simulink model "trajectoryControlAnalysis"  (R2016b)
settings: Solver=VariableStepAuto  StartTime=0.0  StopTime=2  MaxStep=0.01  RelTol=1e-4  EnableMultiTasking=on
values from neighbouring files (symbols this model uses):
  La = 1    [analysis.m]    (also in main.m; purePursuitController.m = 0)
  v = 1    [analysis.m]    (also in main.m = U(1,inode))
undefined symbols (not defined in the file or in its folder): bic, g, gainK
settings Model: Creator=aniket  LastModifiedBy=aniket
settings DataIOCC: LimitDataPoints=on  SaveOutput=off  SaveTime=off
settings OptimizationCC: ExpressionDepthLimit=2147483647  LifeSpan=1
settings DebuggingCC: UnderspecifiedInitializationDetection=Classic  MergeDetectMultiDrivingBlocksExec=none  FcnCallInpInsideContextMsg=warning  AllowSymbolicDim=off  StateNameClashWarn=warning  SFUnexpectedBacktrackingDiag=warning  SFNoUnconditionalDefaultTransitionDiag=warning  SFExecutionAtInitializationDiag=none
settings GRTTargetCC: TargetLangStandard=C89/C90 (ANSI)  GeneratePreprocessorConditionals=Disable all  CombineOutputUpdateFcns=off  GRTInterface=on

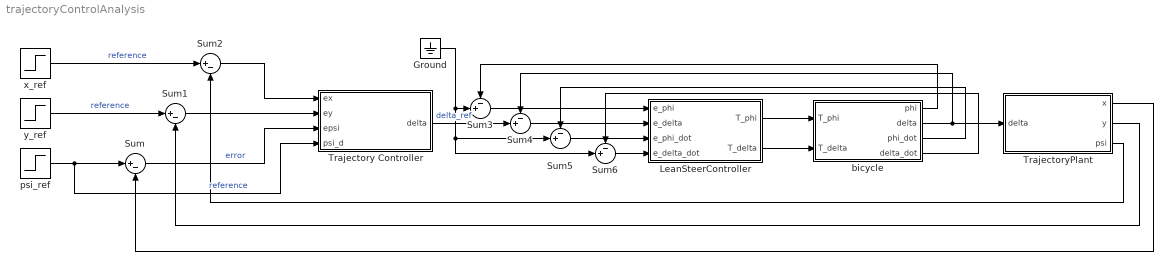
== system trajectoryControlAnalysis ==
  Ground : Ground
  LeanSteerController : Subsystem
  Sum : Sum  Inputs=|+-
  Sum1 : Sum  Inputs=|+-
  Sum2 : Sum  Inputs=|+-
  Sum{3..6} (4 alike) : Sum  Inputs=-+|
  Trajectory Controller : Subsystem
  TrajectoryPlant : Subsystem
  bicycle : Subsystem
  psi_ref : Step  SampleTime=0
  x_ref : Step  SampleTime=0
  y_ref : Step  SampleTime=0
  wires:
  psi_ref/1 -> Trajectory Controller/4(psi_d), Sum/1  "reference"
  TrajectoryPlant/1(x) -> Sum/2
  y_ref/1 -> Sum1/1  "reference"
  x_ref/1 -> Sum2/1  "reference"
  TrajectoryPlant/2(y) -> Sum1/2
  TrajectoryPlant/3(psi) -> Sum2/2
  Sum/1 -> Trajectory Controller/3(epsi)  "error"
  Sum1/1 -> Trajectory Controller/2(ey)
  Sum2/1 -> Trajectory Controller/1(ex)
  LeanSteerController/1(T_phi) -> bicycle/1(T_phi)
  LeanSteerController/2(T_delta) -> bicycle/2(T_delta)
  Sum3/1 -> LeanSteerController/1(e_phi)
  Sum4/1 -> LeanSteerController/2(e_delta)
  Sum5/1 -> LeanSteerController/3(e_phi_dot)
  Sum6/1 -> LeanSteerController/4(e_delta_dot)
  bicycle/1(phi) -> Sum3/1
  bicycle/2(delta) -> TrajectoryPlant/1(delta), Sum4/1
  bicycle/3(phi_dot) -> Sum5/1
  bicycle/4(delta_dot) -> Sum6/1
  Trajectory Controller/1(delta) -> Sum4/2  "delta_ref"
  Ground/1 -> Sum6/2, Sum5/2, Sum3/2

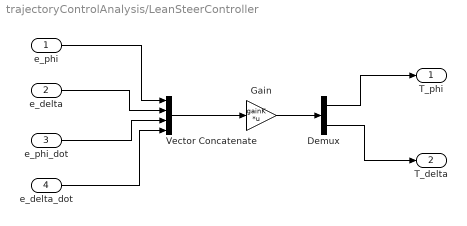
== system trajectoryControlAnalysis/LeanSteerController ==
  e_phi : Inport
  e_delta : Inport  Port=2
  e_phi_dot : Inport  Port=3
  e_delta_dot : Inport  Port=4
  Demux : Demux  Outputs=2
  Gain : Gain  Gain=gainK  Multiplication=Matrix(K*u) (u vector)
  Vector Concatenate : Concatenate  NumInputs=4
  T_phi : Outport
  T_delta : Outport  Port=2
  wires:
  Gain/1 -> Demux/1
  e_phi/1 -> Vector Concatenate/1
  e_delta/1 -> Vector Concatenate/2
  e_phi_dot/1 -> Vector Concatenate/3
  e_delta_dot/1 -> Vector Concatenate/4
  Vector Concatenate/1 -> Gain/1
  Demux/2 -> T_delta/1
  Demux/1 -> T_phi/1

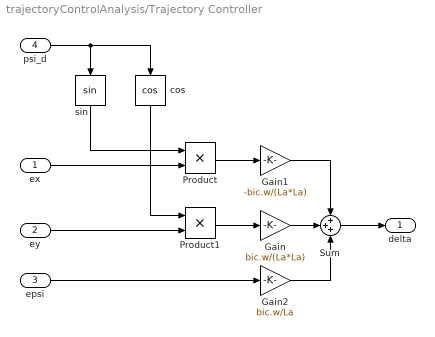
== system trajectoryControlAnalysis/Trajectory Controller ==
  ex : Inport
  ey : Inport  Port=2
  epsi : Inport  Port=3
  psi_d : Inport  Port=4
  Gain : Gain  Gain=bic.w/(La*La)
  Gain1 : Gain  Gain=-bic.w/(La*La)
  Gain2 : Gain  Gain=bic.w/La
  Product : Product
  Product1 : Product
  Sum : Sum  Inputs=+++
  cos : Trigonometry  Operator=cos
  "sin " : Trigonometry
  delta : Outport
  wires:
  Sum/1 -> delta/1
  Gain/1 -> Sum/2
  epsi/1 -> Gain2/1
  Gain1/1 -> Sum/1
  Gain2/1 -> Sum/3
  psi_d/1 -> cos/1, "sin "/1
  Product/1 -> Gain1/1
  Product1/1 -> Gain/1
  ey/1 -> Product1/2
  ex/1 -> Product/2
  "sin "/1 -> Product/1
  cos/1 -> Product1/1

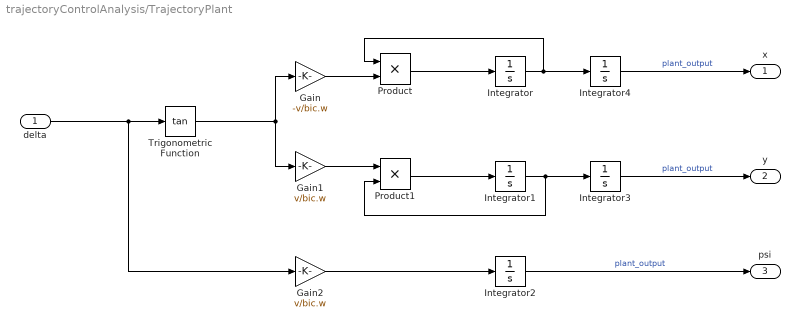
== system trajectoryControlAnalysis/TrajectoryPlant ==
  delta : Inport
  Gain : Gain  Gain=-v/bic.w
  Gain1 : Gain  Gain=v/bic.w
  Gain2 : Gain  Gain=v/bic.w
  Integrator{,1..4} (5 alike) : Integrator
  Product : Product
  Product1 : Product
  Trigonometric Function : Trigonometry  Operator=tan  ApproximationMethod=CORDIC
  x : Outport
  y : Outport  Port=2
  psi : Outport  Port=3
  wires:
  delta/1 -> Gain2/1, Trigonometric Function/1
  Integrator4/1 -> x/1  "plant_output"
  Trigonometric Function/1 -> Gain1/1, Gain/1
  Integrator/1 -> Integrator4/1, Product/1
  Integrator1/1 -> Integrator3/1, Product1/2
  Product/1 -> Integrator/1
  Product1/1 -> Integrator1/1
  Gain/1 -> Product/2
  Gain1/1 -> Product1/1
  Gain2/1 -> Integrator2/1
  Integrator3/1 -> y/1  "plant_output"
  Integrator2/1 -> psi/1  "plant_output"

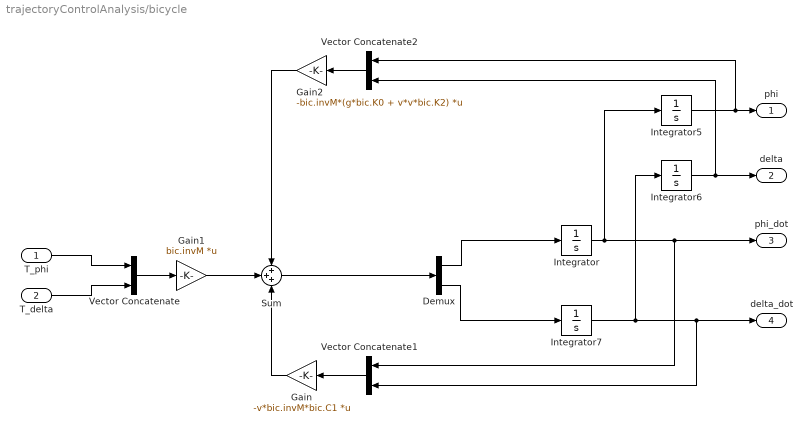
== system trajectoryControlAnalysis/bicycle ==
  T_phi : Inport
  T_delta : Inport  Port=2
  Demux : Demux  Outputs=2
  Gain : Gain  Gain=-v*bic.invM*bic.C1  Multiplication=Matrix(K*u) (u vector)
  Gain1 : Gain  Gain=bic.invM  Multiplication=Matrix(K*u) (u vector)
  Gain2 : Gain  Gain=-bic.invM*(g*bic.K0 + v*v*bic.K2)  Multiplication=Matrix(K*u) (u vector)
  Integrator{,5..7} (4 alike) : Integrator
  Sum : Sum  Inputs=+++
  Vector Concatenate : Concatenate
  Vector Concatenate1 : Concatenate
  Vector Concatenate2 : Concatenate
  phi : Outport
  delta : Outport  Port=2
  phi_dot : Outport  Port=3
  delta_dot : Outport  Port=4
  wires:
  Integrator6/1 -> Vector Concatenate2/2, delta/1
  Integrator/1 -> Integrator5/1, Vector Concatenate1/1, phi_dot/1
  Integrator7/1 -> Integrator6/1, Vector Concatenate1/2, delta_dot/1
  T_delta/1 -> Vector Concatenate/2
  T_phi/1 -> Vector Concatenate/1
  Vector Concatenate/1 -> Gain1/1
  Vector Concatenate1/1 -> Gain/1
  Integrator5/1 -> Vector Concatenate2/1, phi/1
  Vector Concatenate2/1 -> Gain2/1
  Gain1/1 -> Sum/2
  Gain/1 -> Sum/3
  Gain2/1 -> Sum/1
  Sum/1 -> Demux/1
  Demux/1 -> Integrator/1
  Demux/2 -> Integrator7/1
